simulink model "Direct_Motor_Control"  (Simulink 7.5)
settings: Solver=ode45  StartTime=0  StopTime=1  RelTol=1e-3
libraries: simulink x1
settings Model: Creator=lm  LastModifiedBy=lm

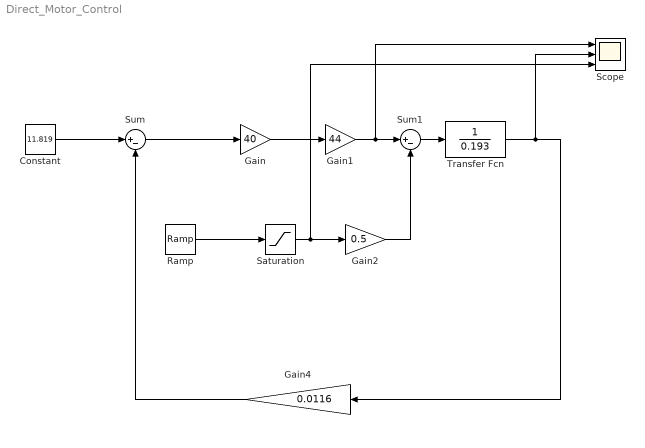
== system Direct_Motor_Control ==
  Constant : Constant  Value=11.819  OutDataType=fixdt(1, 16)  OutScaling=2^0
  Gain : Gain  Gain=40  ParameterDataType=fixdt(1, 16)  ParameterScaling=2^0  OutDataType=fixdt(1, 16)  OutScaling=2^0
  Gain1 : Gain  Gain=44  ParameterDataType=fixdt(1, 16)  ParameterScaling=2^0  OutDataType=fixdt(1, 16)  OutScaling=2^0
  Gain2 : Gain  Gain=0.5  ParameterDataType=fixdt(1, 16)  ParameterScaling=2^0  OutDataType=fixdt(1, 16)  OutScaling=2^0
  Gain4 : Gain  Gain=0.0116  ParameterDataType=fixdt(1, 16)  ParameterScaling=2^0  OutDataType=fixdt(1, 16)  OutScaling=2^0
  Ramp : simulink/Sources/Ramp  SystemSampleTime=-1  slope=100  start=0.1  X0=0
  Saturation : Saturate  UpperLimit=55  OutDataType=fixdt(1, 16)  OutScaling=2^0
  Scope : Scope  NumInputPorts=3
      settings: YMin=-5~-5~-5  YMax=5~5~5
  Sum : Sum  Inputs=|+-  OutDataType=fixdt(1, 16)  OutScaling=2^0
  Sum1 : Sum  Inputs=|+-  OutDataType=fixdt(1, 16)  OutScaling=2^0
  Transfer Fcn : TransferFcn  Denominator=[0 0.193]
  wires:
  Constant/1 -> Sum/1
  Sum/1 -> Gain/1
  Gain/1 -> Gain1/1
  Gain1/1 -> Sum1/1, Scope/1
  Ramp/1 -> Saturation/1
  Saturation/1 -> Gain2/1, Scope/3
  Gain2/1 -> Sum1/2
  Transfer Fcn/1 -> Gain4/1, Scope/2
  Gain4/1 -> Sum/2
  Sum1/1 -> Transfer Fcn/1
